simulink model "BatteryController_empat_PV_WindTurbine_fix1"  (R2015a)
settings: Solver=FixedStepDiscrete  StartTime=0.0  StopTime=10.0  FixedStep=5e-6  RelTol=1e-3
values from neighbouring files (symbols this model uses):
  n = 1500    [ini.m]
  Rs = 2.6e-3    (= 0.0026)    [ini.m]
undefined symbols (not defined in the file or in its folder): Eg0, Ion, Isc, K, ki, Lithium, Ns, q, Rsh, Tn, Voc
libraries: powerlib x56, electricdrivelib x5, re_lib x1
settings Model: Creator=Jodi  LastModifiedBy=David

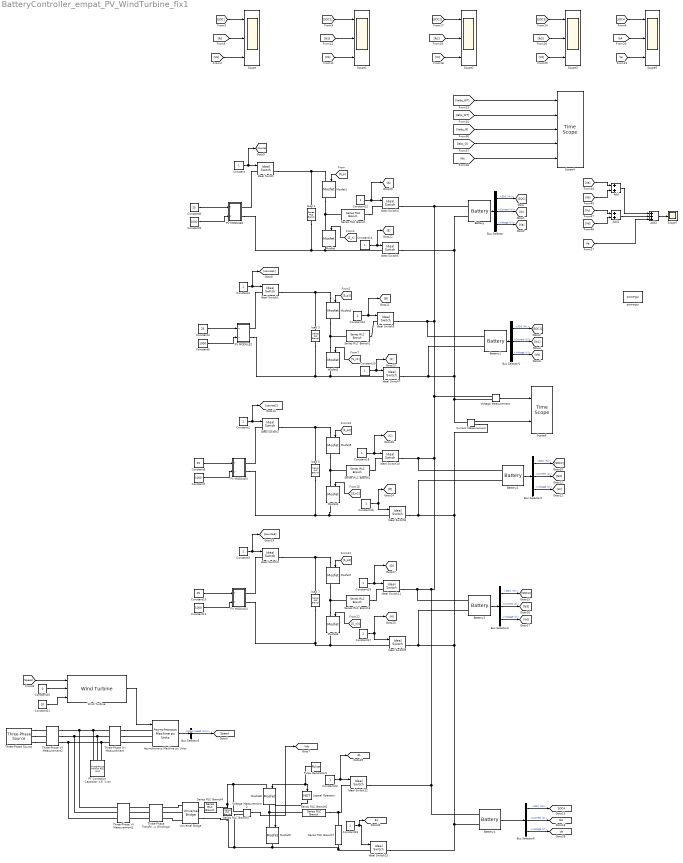
== system BatteryController_empat_PV_WindTurbine_fix1 ==
  Add : Sum
  Add1 : Sum
  Add2 : Sum  Inputs=+++
  Asynchronous Machine pu Units : powerlib/Machines/Asynchronous Machine pu Units  RotorType=Squirrel-cage  PresetModel=No  MechanicalLoad=Torque Tm  ShowDetailedParameters=on  ReferenceFrame=Rotor  Units=pu  MeasurementBus=off  NominalParameters=[400 220 50]  Stator=[0.01965 0.0397]  Rotor=[0.01909 0.0397]  Cage1=[0.01909 0.0397]  Cage2=[0.01909 0.0397]  Lm=1.354  Mechanical=[0.09526 0.05479 2]  PolePairs=2  InitialConditions="[ 1,0   0,0,0   0,0,0 ]"  SimulateSaturation=off  Saturation="[0.212,0.4201,0.8125,1.0979,1.4799,2.2457,3.2586,4.5763,6.4763 ;   0.5,0.7,0.9,1,1.1,1.2 ,1.3,1.4,1.5]"  LoadFlowParameters=0  TsPowergui=0  TsBlock=-1  IterativeModel=Trapezoidal non iterative  Pmec=0
  Battery{,1..3} (4 alike) : electricdrivelib/Extra Sources/Battery  BatType=Lithium-Ion  ShowDetailedParameters=off  NomV=12  NomQ=50  SOC=45  PresetModel=on  MaxQ=50  FullV=13.9678  Dis_rate=21.7391  R=0.0024  Normal_OP=45.2174  expZone="[12.9646      2.45652]"  current=[6.5 13 32.5]  Units=Time  Batt_Tr=1
  Battery4 : electricdrivelib/Extra Sources/Battery  BatType=Lithium-Ion  ShowDetailedParameters=off  NomV=12  NomQ=12  SOC=45  PresetModel=on  MaxQ=12  FullV=13.9678  Dis_rate=5.2174  R=0.01  Normal_OP=10.8522  expZone="[12.9646     0.589565]"  current=[6.5 13 32.5]  Units=Time  Batt_Tr=30
  Bus Selector{,1..3,6} (5 alike) : BusSelector  OutputSignals=SOC (%),Current (A),Voltage (V)
  Bus Selector5 : BusSelector  OutputSignals=Mechanical.Rotor speed (wm)
  Constant{,1..3,12..19,22..23} (14 alike) : Constant
  Constant{4,6,8,10} (4 alike) : Constant  Value=25
  Constant{5,7,9,11} (4 alike) : Constant  Value=1000
  Constant20 : Constant  Value=0
  Constant21 : Constant  Value=10
  Current Measurement : powerlib/Measurements/Current Measurement  PhasorSimulation=off  OutputType=Complex  PSBequivalent=0
  Ideal Switch{,1..13} (14 alike) : powerlib/Power Electronics/Ideal Switch  Ron=0.001  Lon=0  IC=0  Rs=1e5  Cs=inf  Measurements=on
  Logical Operator : Logic  Operator=NOT  AllPortsSameDT=off  OutDataTypeStr=boolean
  Mosfet{,1..7} (8 alike) : powerlib/Power Electronics/Mosfet  Ron=0.1  Lon=0  Rd=0.01  Vfd=0  IC=0  Rs=1e5  Cs=inf  Measurements=on
  Mosfet8 : powerlib/Power Electronics/Mosfet  Ron=0.1  Lon=0  Rd=0.01  Vfd=0  IC=0  Rs=1e5  Cs=inf  Measurements=off
  Mosfet9 : powerlib/Power Electronics/Mosfet  Ron=0.1  Lon=0  Rd=0.01  Vfd=0  IC=0  Rs=1e5  Cs=inf  Measurements=off
  PF Correction Capacitor 1.5  kvar : powerlib/Elements/Three-Phase Parallel RLC Load  LConnTagsString=A|B|C  Configuration=Delta  NominalVoltage=480  NominalFrequency=50  ActivePower=0  InductivePower=0  CapacitivePower=1.5e3  Measurements=None  LoadType=constant Z
  PV MODULE1 : Subsystem
  PV MODULE2 : Subsystem
  PV MODULE3 : Subsystem
  PV MODULE4 : Subsystem
  Pulse Generator3 : DiscretePulseGenerator  PulseType=Time based  Period=10  PulseWidth=5
  Scope{,1..3,5} (5 alike) : Scope  NumInputPorts=3
      Scope settings: TimeRange=10  YMin=42.75~-7.04708e-05~12.2718  YMax=47.25~-7.04704e-05~13.5636  SampleInput=on
      Scope1 settings: TimeRange=10  YMin=42.75~-0.00025~12.2718  YMax=47.25~0~13.5636  SampleInput=on
      Scope2 settings: TimeRange=10  YMin=42.75~0~24.5437  YMax=47.25~4e-05~27.1273  SaveName=ScopeData2  SampleInput=on
      Scope3 settings: TimeRange=10  YMin=42.75~0~24.5437  YMax=47.25~4e-05~27.1273  SaveName=ScopeData3  SampleInput=on
      Scope5 settings: TimeRange=10  YMin=0~-1~0  YMax=100~1~50  SaveName=ScopeData5  SampleInput=on
  Scope4 : TimeScope  NumInputPorts=5
  Scope6 : TimeScope  NumInputPorts=2
  Scope7 : Scope
      settings: YMin=0  YMax=70  SaveName=ScopeData7
  Series RLC Branch{,1..3} (4 alike) : powerlib/Elements/Series RLC Branch  LConnTagsString=__new0  RConnTagsString=__new0  BranchType=RL  Resistance=0.05  Inductance=5.76e-4  SetiL0=off  InitialCurrent=0  Capacitance=1e-6  Setx0=off  InitialVoltage=0  Measurements=None
  Series RLC Branch4 : powerlib/Elements/Series RLC Branch  LConnTagsString=__new0  RConnTagsString=__new0  BranchType=L  Resistance=100  Inductance=1e-3  SetiL0=off  InitialCurrent=0  Capacitance=1e-6  Setx0=off  InitialVoltage=0  Measurements=None
  Series RLC Branch5 : powerlib/Elements/Series RLC Branch  LConnTagsString=__new0  RConnTagsString=__new0  BranchType=C  Resistance=100  Inductance=1e-3  SetiL0=off  InitialCurrent=0  Capacitance=1e-3  Setx0=off  InitialVoltage=0  Measurements=None
  Series RLC Branch6 : powerlib/Elements/Series RLC Branch  LConnTagsString=__new0  RConnTagsString=__new0  BranchType=RL  Resistance=100  Inductance=1e-3  SetiL0=off  InitialCurrent=0  Capacitance=1e-6  Setx0=off  InitialVoltage=0  Measurements=None
  Series RLC Branch7 : powerlib/Elements/Series RLC Branch  LConnTagsString=__new0  RConnTagsString=__new0  BranchType=RC  Resistance=100  Inductance=1e-3  SetiL0=off  InitialCurrent=0  Capacitance=1e-6  Setx0=off  InitialVoltage=0  Measurements=None
  Three-Phase Transformer (Two Windings) : powerlib/Elements/Three-Phase Transformer (Two Windings)  Winding1Connection=Yg  Winding2Connection=Yg  CoreType=Three single-phase transformers  SetSaturation=off  Hysteresis=off  DataFile='hysteresis'  SetInitialFlux=off  Measurements=None  UNITS=pu  NominalPower=[ 250e6 , 50 ]  Winding1=[ 735e3 , 0.002 , 0.08 ]  Winding2=[ 315e3 , 0.002 , 0.08 ]  Rm=100  Lm=500  L0=0.5  Saturation=[ 0,0 ; 0.0024,1.2 ; 1.0,1.52 ]  InitialFluxes=[ 0.8 , -0.8 , 0.7 ]  MoreParameters=off  BreakLoop=off  DataType=off  TransfoNumber=1
  Three-Phase V-I Measurement : powerlib/Measurements/Three-Phase V-I Measurement  VoltageMeasurement=phase-to-ground  SetLabelV=on  LabelV=Vabc_WT  Vpu=off  VpuLL=off  CurrentMeasurement=yes  SetLabelI=on  LabelI=Iabc_WT  Ipu=off  Pbase=100e6  Vbase=500e3  OutputType=Complex  PhasorSimulation=off  PSBequivalent=0
  Three-Phase V-I Measurement1 : powerlib/Measurements/Three-Phase V-I Measurement  VoltageMeasurement=phase-to-phase  SetLabelV=on  LabelV=Vabc_G  Vpu=off  VpuLL=off  CurrentMeasurement=yes  SetLabelI=on  LabelI=Iabc_G  Ipu=off  Pbase=100e6  Vbase=500e3  OutputType=Complex  PhasorSimulation=off  PSBequivalent=0
  Three-Phase V-I Measurement2 : powerlib/Measurements/Three-Phase V-I Measurement  VoltageMeasurement=phase-to-ground  SetLabelV=on  LabelV=Vabc_SC  Vpu=off  VpuLL=off  CurrentMeasurement=yes  SetLabelI=on  LabelI=Iabc_SC  Ipu=off  Pbase=100e6  Vbase=500e3  OutputType=Complex  PhasorSimulation=off  PSBequivalent=0
  Three-Phase Source : powerlib/Electrical Sources/Three-Phase Source  Voltage=220  PhaseAngle=4  Frequency=50  InternalConnection=Yg  SpecifyImpedance=on  Resistance=0.8929  Inductance=16.58e-3  ShortCircuitLevel=100e6  BaseVoltage=25e3  XRratio=7  BusType=swing  Pref=0  Qref=0  Qmin=-inf  Qmax=inf
  Universal Bridge : powerlib/Power Electronics/Universal Bridge  Arms=3  SnubberResistance=100  SnubberCapacitance=inf  Device=Diodes  Ron=1e-3  Lon=0  ForwardVoltages="[  0  0  ]"  ForwardVoltage=0  GTOparameters=[ 10e-6 , 20e-6 ]  IGBTparameters=[ 1e-6 , 2e-6 ]  Measurements=None  Measurements_2=None  converterType=Rectifier
  Voltage Measurement : powerlib/Measurements/Voltage Measurement  PhasorSimulation=off  OutputType=Complex  PSBequivalent=0
  Voltage Measurement2 : powerlib/Measurements/Voltage Measurement  PhasorSimulation=off  OutputType=Complex  PSBequivalent=0
  Wind Turbine : re_lib/Wind Generation/Wind Turbine  Pnom=400  Pelec_base=400/0.9  wind_base=12  P_wind_base=0.73  speed_nom=1.2  pitch_angle=0  c1_c6="[0.51763          116          0.4            5           21     0.006795]"  cp_nom=0.48  lambda_nom=8.1
  load {1,3,5,7} (4 alike) : powerlib/Elements/Series RLC Branch  LConnTagsString=__new0  RConnTagsString=__new0  BranchType=RC  Resistance=0.001  Inductance=5.76e-4  SetiL0=off  InitialCurrent=0  Capacitance=1000e-6  Setx0=off  InitialVoltage=0  Measurements=None
  powergui : powerlib/powergui  Priority=1  SimulationMode=Discrete  SolverType=Tustin/Backward Euler (TBE)  SampleTime=5e-06  frequency=60  SPID=off  DisableSnubberDevices=off  DisableRonSwitches=off  DisableVfSwitches=off  SwTol=0  DisplayEquations=off  Interpol=off  methode=off  Ts=100  FunctionMessages=off  echomessages=off  HookPort=off  EnableUseOfTLC=off  x0status=blocks  frequencyindice=0  Pbase=100e6  ErrMax=1e-4  Iterations=50  UnitsV=kV  UnitsW=MW  buscounter=0  RestoreLinks=warning  ResistiveCurrentMeasurement=off  Frange=[0:2:500]  Ylog=off  Xlog=on  ShowGrid=off  save=off  variable=ZData  structure=0  ZoomFFT=off  StartTime=0.0  cycles=1  DisplayStyle=1  fundamental=60  FreqAxis=off  MaxFrequency=1000  frequencyindicesteady=1  RmsSteady=1  display=off
  tag scope: A1=global, E1=global, Ib4=global, SOC4=global, Speed=global, Vdc=global, Ve=global
  wires:
  Constant/1 -> [source], Ideal Switch/1
  Battery/1 -> Bus Selector/1
  Bus Selector/1 -> [SOC]  "<SOC (%)>"
  Bus Selector/2 -> [Ib]  "<Current (A)>"
  Bus Selector/3 -> [Va]  "<Voltage (V)>"
  [S_p] -> Mosfet1/1
  [S_n] -> Mosfet/1
  [SOC] -> Scope/1
  [Va] -> Scope/3
  Constant1/1 -> [source1], Ideal Switch1/1
  Battery1/1 -> Bus Selector1/1
  Bus Selector1/1 -> [SOC1]  "<SOC (%)>"
  Bus Selector1/2 -> [Ib1]  "<Current (A)>"
  Bus Selector1/3 -> [Vb]  "<Voltage (V)>"
  [S_p1] -> Mosfet3/1
  [S_n1] -> Mosfet2/1
  [SOC1] -> Scope1/1
  [Vb] -> Scope1/3
  Constant2/1 -> [source2], Ideal Switch2/1
  Battery2/1 -> Bus Selector2/1
  Bus Selector2/1 -> [SOC2]  "<SOC (%)>"
  Bus Selector2/2 -> [Ib2]  "<Current (A)>"
  Bus Selector2/3 -> [Vc]  "<Voltage (V)>"
  [S_p2] -> Mosfet5/1
  [S_n2] -> Mosfet4/1
  [SOC2] -> Scope2/1
  [Vc] -> Scope2/3
  Constant3/1 -> [source3], Ideal Switch3/1
  Battery3/1 -> Bus Selector3/1
  Bus Selector3/1 -> [SOC3]  "<SOC (%)>"
  Bus Selector3/2 -> [Ib3]  "<Current (A)>"
  Bus Selector3/3 -> [Vd]  "<Voltage (V)>"
  [S_p3] -> Mosfet7/1
  [S_n3] -> Mosfet6/1
  [SOC3] -> Scope3/1
  [Vd] -> Scope3/3
  Constant8/1 -> PV MODULE1/1(T)
  Constant9/1 -> PV MODULE1/2(Ir)
  Constant4/1 -> PV MODULE2/1(T)
  Constant5/1 -> PV MODULE2/2(Ir)
  Constant6/1 -> PV MODULE3/1(T)
  Constant7/1 -> PV MODULE3/2(Ir)
  Constant10/1 -> PV MODULE4/1(T)
  Constant11/1 -> PV MODULE4/2(Ir)
  Constant12/1 -> [A], Ideal Switch4/1
  Constant13/1 -> [B], Ideal Switch5/1
  Constant14/1 -> [E], Ideal Switch6/1
  Constant15/1 -> Ideal Switch7/1, [F]
  Constant16/1 -> [G], Ideal Switch8/1
  Constant17/1 -> [H], Ideal Switch9/1
  Constant18/1 -> [C], Ideal Switch10/1
  Constant19/1 -> [D], Ideal Switch11/1
  Wind Turbine/1 -> Asynchronous Machine pu Units/1
  Asynchronous Machine pu Units/1 -> Bus Selector5/1
  Bus Selector5/1 -> [Speed]  "<Rotor speed (wm)>"
  [Speed] -> Wind Turbine/1
  Constant20/1 -> Wind Turbine/2
  Constant21/1 -> Wind Turbine/3
  Battery4/1 -> Bus Selector6/1
  Pulse Generator3/1 -> Logical Operator/1, Mosfet8/1
  Logical Operator/1 -> Mosfet9/1
  Voltage Measurement2/1 -> [Vdc]
  Bus Selector6/1 -> [SOC4]  "<SOC (%)>"
  Bus Selector6/2 -> [Ib4]  "<Current (A)>"
  Bus Selector6/3 -> [Ve]  "<Voltage (V)>"
  [Vabc_WT] -> Scope4/1
  [Iabc_G] -> Scope4/4
  [Vabc_G] -> Scope4/3
  [Iabc_WT] -> Scope4/2
  [Vdc] -> Scope4/5
  Constant22/1 -> [A1], Ideal Switch12/1
  Constant23/1 -> [E1], Ideal Switch13/1
  [Ib] -> Scope/2
  [Ib1] -> Scope1/2
  [Ib2] -> Scope2/2
  [Ib3] -> Scope3/2
  [SOC4] -> Scope5/1
  [Ve] -> Scope5/3
  [Ib4] -> Scope5/2
  [Va] -> Add/1
  [Vb] -> Add/2
  [Vc] -> Add1/1
  [Vd] -> Add1/2
  Add/1 -> Add2/1
  Add1/1 -> Add2/2
  Add2/1 -> Scope7/1
  [Ve] -> Add2/3
  Current Measurement/1 -> Scope6/2
  Voltage Measurement/1 -> Scope6/1
  connections:
  Mosfet1/RConn1 -- Series RLC Branch/LConn1 -- Mosfet/LConn1
  PV MODULE1/RConn2 -- load 1/RConn1 -- Ideal Switch6/LConn1 -- Mosfet/RConn1
  load 1/LConn1 -- Ideal Switch/RConn1 -- Mosfet1/LConn1
  Ideal Switch/LConn1 -- PV MODULE1/RConn1
  Mosfet2/LConn1 -- Mosfet3/RConn1 -- Series RLC Branch1/LConn1
  load 3/RConn1 -- PV MODULE2/RConn2 -- Mosfet2/RConn1 -- Ideal Switch7/LConn1
  Mosfet3/LConn1 -- Ideal Switch1/RConn1 -- load 3/LConn1
  Ideal Switch1/LConn1 -- PV MODULE2/RConn1
  Mosfet4/LConn1 -- Mosfet5/RConn1 -- Series RLC Branch2/LConn1
  load 5/RConn1 -- PV MODULE3/RConn2 -- Mosfet4/RConn1 -- Ideal Switch8/LConn1
  Mosfet5/LConn1 -- Ideal Switch2/RConn1 -- load 5/LConn1
  Ideal Switch2/LConn1 -- PV MODULE3/RConn1
  Mosfet6/LConn1 -- Mosfet7/RConn1 -- Series RLC Branch3/LConn1
  load 7/RConn1 -- PV MODULE4/RConn2 -- Ideal Switch9/LConn1 -- Mosfet6/RConn1
  Mosfet7/LConn1 -- Ideal Switch3/RConn1 -- load 7/LConn1
  Ideal Switch3/LConn1 -- PV MODULE4/RConn1
  Series RLC Branch/RConn1 -- Ideal Switch4/LConn1
  Ideal Switch5/LConn1 -- Series RLC Branch1/RConn1
  Series RLC Branch2/RConn1 -- Ideal Switch10/LConn1
  Series RLC Branch3/RConn1 -- Ideal Switch11/LConn1
  PF Correction Capacitor 1.5  kvar/LConn1 -- Three-Phase V-I Measurement/RConn1 -- Three-Phase V-I Measurement1/LConn1 -- Three-Phase V-I Measurement2/RConn1
  PF Correction Capacitor 1.5  kvar/LConn2 -- Three-Phase V-I Measurement/RConn2 -- Three-Phase V-I Measurement1/LConn2 -- Three-Phase V-I Measurement2/RConn2
  PF Correction Capacitor 1.5  kvar/LConn3 -- Three-Phase V-I Measurement/RConn3 -- Three-Phase V-I Measurement1/LConn3 -- Three-Phase V-I Measurement2/RConn3
  Series RLC Branch5/LConn1 -- Voltage Measurement2/LConn1 -- Mosfet8/LConn1 -- Series RLC Branch4/RConn1
  Series RLC Branch6/LConn1 -- Mosfet8/RConn1 -- Mosfet9/LConn1
  Series RLC Branch5/RConn1 -- Ideal Switch13/LConn1 -- Series RLC Branch7/RConn1 -- Mosfet9/RConn1 -- Voltage Measurement2/LConn2 -- Universal Bridge/RConn2
  Three-Phase V-I Measurement/LConn1 -- Asynchronous Machine pu Units/LConn1
  Three-Phase V-I Measurement/LConn3 -- Asynchronous Machine pu Units/LConn3
  Three-Phase V-I Measurement/LConn2 -- Asynchronous Machine pu Units/LConn2
  Universal Bridge/LConn3 -- Three-Phase Transformer (Two Windings)/RConn3
  Three-Phase Transformer (Two Windings)/LConn2 -- Three-Phase V-I Measurement1/RConn2
  Universal Bridge/LConn1 -- Three-Phase Transformer (Two Windings)/RConn1
  Three-Phase Transformer (Two Windings)/LConn1 -- Three-Phase V-I Measurement1/RConn1
  Universal Bridge/LConn2 -- Three-Phase Transformer (Two Windings)/RConn2
  Series RLC Branch4/LConn1 -- Universal Bridge/RConn1
  Three-Phase Transformer (Two Windings)/LConn3 -- Three-Phase V-I Measurement1/RConn3
  Series RLC Branch6/RConn1 -- Series RLC Branch7/LConn1 -- Ideal Switch12/LConn1
  Three-Phase Source/RConn1 -- Three-Phase V-I Measurement2/LConn1
  Three-Phase Source/RConn2 -- Three-Phase V-I Measurement2/LConn2
  Three-Phase Source/RConn3 -- Three-Phase V-I Measurement2/LConn3
  Battery4/LConn1 -- Ideal Switch12/RConn1 -- Battery3/LConn1 -- Ideal Switch11/RConn1 -- Battery2/LConn1 -- Ideal Switch10/RConn1 -- Ideal Switch5/RConn1 -- Battery1/LConn1 -- Ideal Switch4/RConn1 -- Battery/LConn1 -- Voltage Measurement/LConn1
  Battery/LConn2 -- Ideal Switch6/RConn1 -- Ideal Switch7/RConn1 -- Battery1/LConn2 -- Current Measurement/LConn1 -- Voltage Measurement/LConn2
  Ideal Switch13/RConn1 -- Battery3/LConn2 -- Ideal Switch9/RConn1 -- Battery2/LConn2 -- Ideal Switch8/RConn1 -- Current Measurement/RConn1 -- Battery4/LConn2

== system BatteryController_empat_PV_WindTurbine_fix1/PV MODULE1 ==
  T : Inport
  Ir : Inport  Port=2
  Controlled Current Source : powerlib/Electrical Sources/Controlled Current Source  Initialize=on  Source_Type=AC  Amplitude=0  Phase=0  Frequency=0  Measurements=None
  PV Module : Subsystem  InitFcn=|
      | ki=.0032,
      | q=1.6e-19,
      | K=1.38e-23,
      | n=1.3,
      | Eg0=1.1,
      | Rs=.221,
      | Rsh=415.405,
      | Tn=298,
      | 
      | Voc=32.9,
      | Isc=8.21,
      | Ns=54,
  Voltage Measurement : powerlib/Measurements/Voltage Measurement  PhasorSimulation=off  OutputType=Complex  PSBequivalent=0
  + : PMIOPort  Port=1  Side=Right
  - : PMIOPort  Port=2  Side=Right
  wires:
  Voltage Measurement/1 -> PV Module/3(V_Array)
  PV Module/1(I) -> Controlled Current Source/1
  Ir/1 -> PV Module/2(G)
  T/1 -> PV Module/1(T)
  connections:
  Controlled Current Source/RConn1 -- +/RConn1 -- Voltage Measurement/LConn1
  Controlled Current Source/LConn1 -- -/RConn1 -- Voltage Measurement/LConn2

== system BatteryController_empat_PV_WindTurbine_fix1/PV MODULE2 ==
  T : Inport
  Ir : Inport  Port=2
  Controlled Current Source : powerlib/Electrical Sources/Controlled Current Source  Initialize=on  Source_Type=AC  Amplitude=0  Phase=0  Frequency=0  Measurements=None
  PV Module : Subsystem  InitFcn=|
      | ki=.0032,
      | q=1.6e-19,
      | K=1.38e-23,
      | n=1.3,
      | Eg0=1.1,
      | Rs=.221,
      | Rsh=415.405,
      | Tn=298,
      | 
      | Voc=32.9,
      | Isc=8.21,
      | Ns=54,
  Voltage Measurement : powerlib/Measurements/Voltage Measurement  PhasorSimulation=off  OutputType=Complex  PSBequivalent=0
  + : PMIOPort  Port=1  Side=Right
  - : PMIOPort  Port=2  Side=Right
  wires:
  Voltage Measurement/1 -> PV Module/3(V_Array)
  PV Module/1(I) -> Controlled Current Source/1
  Ir/1 -> PV Module/2(G)
  T/1 -> PV Module/1(T)
  connections:
  Controlled Current Source/RConn1 -- +/RConn1 -- Voltage Measurement/LConn1
  Controlled Current Source/LConn1 -- -/RConn1 -- Voltage Measurement/LConn2

== system BatteryController_empat_PV_WindTurbine_fix1/PV MODULE3 ==
  T : Inport
  Ir : Inport  Port=2
  Controlled Current Source : powerlib/Electrical Sources/Controlled Current Source  Initialize=on  Source_Type=AC  Amplitude=0  Phase=0  Frequency=0  Measurements=None
  PV Module : Subsystem  InitFcn=|
      | ki=.0032,
      | q=1.6e-19,
      | K=1.38e-23,
      | n=1.3,
      | Eg0=1.1,
      | Rs=.221,
      | Rsh=415.405,
      | Tn=298,
      | 
      | Voc=32.9,
      | Isc=8.21,
      | Ns=54,
  Voltage Measurement : powerlib/Measurements/Voltage Measurement  PhasorSimulation=off  OutputType=Complex  PSBequivalent=0
  + : PMIOPort  Port=1  Side=Right
  - : PMIOPort  Port=2  Side=Right
  wires:
  Voltage Measurement/1 -> PV Module/3(V_Array)
  PV Module/1(I) -> Controlled Current Source/1
  Ir/1 -> PV Module/2(G)
  T/1 -> PV Module/1(T)
  connections:
  Controlled Current Source/RConn1 -- +/RConn1 -- Voltage Measurement/LConn1
  Controlled Current Source/LConn1 -- -/RConn1 -- Voltage Measurement/LConn2

== system BatteryController_empat_PV_WindTurbine_fix1/PV MODULE4 ==
  T : Inport
  Ir : Inport  Port=2
  Controlled Current Source : powerlib/Electrical Sources/Controlled Current Source  Initialize=on  Source_Type=AC  Amplitude=0  Phase=0  Frequency=0  Measurements=None
  PV Module : Subsystem  InitFcn=|
      | ki=.0032,
      | q=1.6e-19,
      | K=1.38e-23,
      | n=1.3,
      | Eg0=1.1,
      | Rs=.221,
      | Rsh=415.405,
      | Tn=298,
      | 
      | Voc=32.9,
      | Isc=8.21,
      | Ns=54,
  Voltage Measurement : powerlib/Measurements/Voltage Measurement  PhasorSimulation=off  OutputType=Complex  PSBequivalent=0
  + : PMIOPort  Port=1  Side=Right
  - : PMIOPort  Port=2  Side=Right
  wires:
  Voltage Measurement/1 -> PV Module/3(V_Array)
  PV Module/1(I) -> Controlled Current Source/1
  Ir/1 -> PV Module/2(G)
  T/1 -> PV Module/1(T)
  connections:
  Controlled Current Source/RConn1 -- +/RConn1 -- Voltage Measurement/LConn1
  Controlled Current Source/LConn1 -- -/RConn1 -- Voltage Measurement/LConn2

== system BatteryController_empat_PV_WindTurbine_fix1/PV MODULE1/PV Module ==
  T : Inport
  G : Inport  Port=2
  V_Array : Inport  Port=3
  Add1 : Sum
  Constant1 : Constant  Value=273
  Photo Current : Subsystem
  Pv Current : Subsystem
  Reverse Saturation Current : Subsystem
  Saturation Current : Subsystem
  Shunt Current : Subsystem
  I : Outport
  wires:
  Pv Current/1(I) -> I/1, Shunt Current/2(I)
  Photo Current/1(Iph) -> Pv Current/4(Iph)
  Saturation Current/1(IO) -> Pv Current/3(IO)
  V_Array/1 -> Shunt Current/1(V), Pv Current/1(V)
  T/1 -> Add1/1
  G/1 -> Photo Current/2(G)
  Reverse Saturation Current/1(Irs) -> Saturation Current/2(Irs)
  Shunt Current/1(Ish) -> Pv Current/5(Ish)
  Constant1/1 -> Add1/2
  Add1/1 -> Saturation Current/1(T), Photo Current/1(T), Reverse Saturation Current/1(T), Pv Current/2(T)

== system BatteryController_empat_PV_WindTurbine_fix1/PV MODULE2/PV Module ==
  T : Inport
  G : Inport  Port=2
  V_Array : Inport  Port=3
  Add1 : Sum
  Constant1 : Constant  Value=273
  Photo Current : Subsystem
  Pv Current : Subsystem
  Reverse Saturation Current : Subsystem
  Saturation Current : Subsystem
  Shunt Current : Subsystem
  I : Outport
  wires:
  Pv Current/1(I) -> I/1, Shunt Current/2(I)
  Photo Current/1(Iph) -> Pv Current/4(Iph)
  Saturation Current/1(IO) -> Pv Current/3(IO)
  V_Array/1 -> Shunt Current/1(V), Pv Current/1(V)
  T/1 -> Add1/1
  G/1 -> Photo Current/2(G)
  Reverse Saturation Current/1(Irs) -> Saturation Current/2(Irs)
  Shunt Current/1(Ish) -> Pv Current/5(Ish)
  Constant1/1 -> Add1/2
  Add1/1 -> Saturation Current/1(T), Photo Current/1(T), Reverse Saturation Current/1(T), Pv Current/2(T)

== system BatteryController_empat_PV_WindTurbine_fix1/PV MODULE3/PV Module ==
  T : Inport
  G : Inport  Port=2
  V_Array : Inport  Port=3
  Add1 : Sum
  Constant1 : Constant  Value=273
  Photo Current : Subsystem
  Pv Current : Subsystem
  Reverse Saturation Current : Subsystem
  Saturation Current : Subsystem
  Shunt Current : Subsystem
  I : Outport
  wires:
  Pv Current/1(I) -> I/1, Shunt Current/2(I)
  Photo Current/1(Iph) -> Pv Current/4(Iph)
  Saturation Current/1(IO) -> Pv Current/3(IO)
  V_Array/1 -> Shunt Current/1(V), Pv Current/1(V)
  T/1 -> Add1/1
  G/1 -> Photo Current/2(G)
  Reverse Saturation Current/1(Irs) -> Saturation Current/2(Irs)
  Shunt Current/1(Ish) -> Pv Current/5(Ish)
  Constant1/1 -> Add1/2
  Add1/1 -> Saturation Current/1(T), Photo Current/1(T), Reverse Saturation Current/1(T), Pv Current/2(T)

== system BatteryController_empat_PV_WindTurbine_fix1/PV MODULE4/PV Module ==
  T : Inport
  G : Inport  Port=2
  V_Array : Inport  Port=3
  Add1 : Sum
  Constant1 : Constant  Value=273
  Photo Current : Subsystem
  Pv Current : Subsystem
  Reverse Saturation Current : Subsystem
  Saturation Current : Subsystem
  Shunt Current : Subsystem
  I : Outport
  wires:
  Pv Current/1(I) -> I/1, Shunt Current/2(I)
  Photo Current/1(Iph) -> Pv Current/4(Iph)
  Saturation Current/1(IO) -> Pv Current/3(IO)
  V_Array/1 -> Shunt Current/1(V), Pv Current/1(V)
  T/1 -> Add1/1
  G/1 -> Photo Current/2(G)
  Reverse Saturation Current/1(Irs) -> Saturation Current/2(Irs)
  Shunt Current/1(Ish) -> Pv Current/5(Ish)
  Constant1/1 -> Add1/2
  Add1/1 -> Saturation Current/1(T), Photo Current/1(T), Reverse Saturation Current/1(T), Pv Current/2(T)

== system BatteryController_empat_PV_WindTurbine_fix1/PV MODULE1/PV Module/Photo Current ==
  note: Iph=[Isc + {ki*(T-298)}]*G/1000
  T : Inport
  G : Inport  Port=2
  Add1 : Sum  Inputs=+-
  Add2 : Sum  Inputs=+-
  Constant1 : Constant  Value=298
  Constant2 : Constant  Value=ki
  Constant3 : Constant  Value=Isc
  Constant4 : Constant  Value=1000
  Product1 : Product
  Product2 : Product
  Product3 : Product  Inputs=*/
  Iph : Outport
  wires:
  Add2/1 -> Product2/2
  Product3/1 -> Iph/1
  Constant4/1 -> Product3/2
  Constant1/1 -> Add1/2
  Product2/1 -> Product3/1
  G/1 -> Product2/1
  Constant2/1 -> Product1/2
  Product1/1 -> Add2/2
  Add1/1 -> Product1/1
  T/1 -> Add1/1
  Constant3/1 -> Add2/1

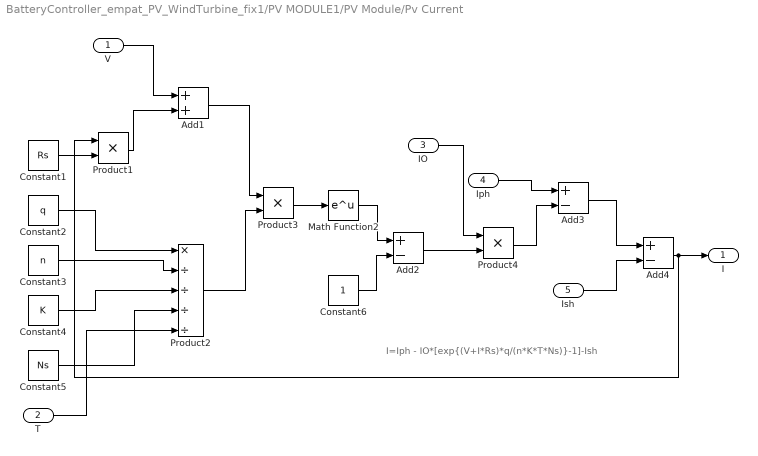
== system BatteryController_empat_PV_WindTurbine_fix1/PV MODULE1/PV Module/Pv Current ==
  note: I=Iph - IO*[exp{(V+I*Rs)*q/(n*K*T*Ns)}-1]-Ish
  V : Inport
  T : Inport  Port=2
  IO : Inport  Port=3
  Iph : Inport  Port=4
  Ish : Inport  Port=5
  Add1 : Sum
  Add2 : Sum  Inputs=+-
  Add3 : Sum  Inputs=+-
  Add4 : Sum  Inputs=+-
  Constant1 : Constant  Value=Rs
  Constant2 : Constant  Value=q
  Constant3 : Constant  Value=n
  Constant4 : Constant  Value=K
  Constant5 : Constant  Value=Ns
  Constant6 : Constant
  Math Function2 : Math  SaturateOnIntegerOverflow=on
  Product1 : Product
  Product2 : Product  Inputs=*////
  Product3 : Product
  Product4 : Product
  I : Outport
  wires:
  Constant3/1 -> Product2/2
  Constant4/1 -> Product2/3
  Add2/1 -> Product4/2
  Add3/1 -> Add4/1
  Constant5/1 -> Product2/4
  Iph/1 -> Add3/1
  Product1/1 -> Add1/2
  Product2/1 -> Product3/2
  T/1 -> Product2/5
  Product3/1 -> Math Function2/1
  Math Function2/1 -> Add2/1
  Add1/1 -> Product3/1
  Constant2/1 -> Product2/1
  V/1 -> Add1/1
  IO/1 -> Product4/1
  Constant6/1 -> Add2/2
  Ish/1 -> Add4/2
  Add4/1 -> I/1, Product1/1
  Product4/1 -> Add3/2
  Constant1/1 -> Product1/2

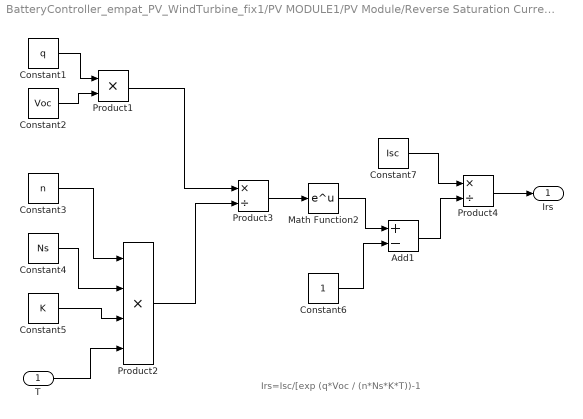
== system BatteryController_empat_PV_WindTurbine_fix1/PV MODULE1/PV Module/Reverse Saturation Current ==
  note: Irs=Isc/[exp (q*Voc / (n*Ns*K*T))-1
  T : Inport
  Add1 : Sum  Inputs=+-
  Constant1 : Constant  Value=q
  Constant2 : Constant  Value=Voc
  Constant3 : Constant  Value=n
  Constant4 : Constant  Value=Ns
  Constant5 : Constant  Value=K
  Constant6 : Constant
  Constant7 : Constant  Value=Isc
  Math Function2 : Math  SaturateOnIntegerOverflow=on
  Product1 : Product
  Product2 : Product  Inputs=4
  Product3 : Product  Inputs=*/
  Product4 : Product  Inputs=*/
  Irs : Outport
  wires:
  Product4/1 -> Irs/1
  Constant1/1 -> Product1/1
  Math Function2/1 -> Add1/1
  Constant6/1 -> Add1/2
  Constant3/1 -> Product2/1
  Add1/1 -> Product4/2
  Product2/1 -> Product3/2
  Constant7/1 -> Product4/1
  Product3/1 -> Math Function2/1
  Product1/1 -> Product3/1
  Constant2/1 -> Product1/2
  T/1 -> Product2/4
  Constant5/1 -> Product2/3
  Constant4/1 -> Product2/2

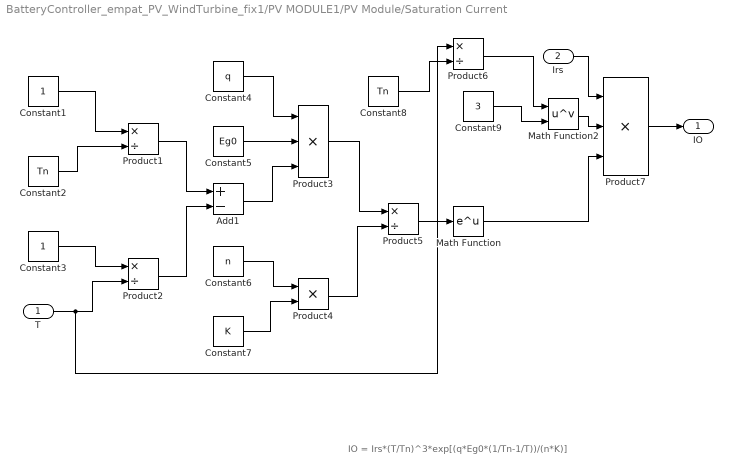
== system BatteryController_empat_PV_WindTurbine_fix1/PV MODULE1/PV Module/Saturation Current ==
  note: IO = Irs*(T/Tn)^3*exp[(q*Eg0*(1/Tn-1/T))/(n*K)]
  T : Inport
  Irs : Inport  Port=2
  Add1 : Sum  Inputs=+-
  Constant1 : Constant
  Constant2 : Constant  Value=Tn
  Constant3 : Constant
  Constant4 : Constant  Value=q
  Constant5 : Constant  Value=Eg0
  Constant6 : Constant  Value=n
  Constant7 : Constant  Value=K
  Constant8 : Constant  Value=Tn
  Constant9 : Constant  Value=3
  Math Function : Math  SaturateOnIntegerOverflow=on
  Math Function2 : Math  Operator=pow  SaturateOnIntegerOverflow=on
  Product{1..2,5..6} (4 alike) : Product  Inputs=*/
  Product3 : Product  Inputs=3
  Product4 : Product
  Product7 : Product  Inputs=3
  IO : Outport
  wires:
  Product7/1 -> IO/1
  Product4/1 -> Product5/2
  Product5/1 -> Math Function/1
  Math Function2/1 -> Product7/2
  Constant2/1 -> Product1/2
  Add1/1 -> Product3/3
  Constant5/1 -> Product3/2
  Constant7/1 -> Product4/2
  Constant4/1 -> Product3/1
  Constant8/1 -> Product6/2
  Product2/1 -> Add1/2
  T/1 -> Product6/1, Product2/2
  Constant1/1 -> Product1/1
  Math Function/1 -> Product7/3
  Product6/1 -> Math Function2/1
  Constant9/1 -> Math Function2/2
  Irs/1 -> Product7/1
  Constant3/1 -> Product2/1
  Product3/1 -> Product5/1
  Constant6/1 -> Product4/1
  Product1/1 -> Add1/1

== system BatteryController_empat_PV_WindTurbine_fix1/PV MODULE1/PV Module/Shunt Current ==
  note: Ish=(V+I*Rs)/Rsh
  V : Inport
  I : Inport  Port=2
  Add1 : Sum
  Constant1 : Constant  Value=Rs
  Constant2 : Constant  Value=Rsh
  Product1 : Product  Inputs=**
  Product2 : Product  Inputs=*/
  Ish : Outport
  wires:
  I/1 -> Product1/1
  Constant1/1 -> Product1/2
  Constant2/1 -> Product2/2
  Add1/1 -> Product2/1
  Product1/1 -> Add1/1
  Product2/1 -> Ish/1
  V/1 -> Add1/2

== system BatteryController_empat_PV_WindTurbine_fix1/PV MODULE2/PV Module/Photo Current ==
  note: Iph=[Isc + {ki*(T-298)}]*G/1000
  T : Inport
  G : Inport  Port=2
  Add1 : Sum  Inputs=+-
  Add2 : Sum  Inputs=+-
  Constant1 : Constant  Value=298
  Constant2 : Constant  Value=ki
  Constant3 : Constant  Value=Isc
  Constant4 : Constant  Value=1000
  Product1 : Product
  Product2 : Product
  Product3 : Product  Inputs=*/
  Iph : Outport
  wires:
  Add2/1 -> Product2/2
  Product3/1 -> Iph/1
  Constant4/1 -> Product3/2
  Constant1/1 -> Add1/2
  Product2/1 -> Product3/1
  G/1 -> Product2/1
  Constant2/1 -> Product1/2
  Product1/1 -> Add2/2
  Add1/1 -> Product1/1
  T/1 -> Add1/1
  Constant3/1 -> Add2/1

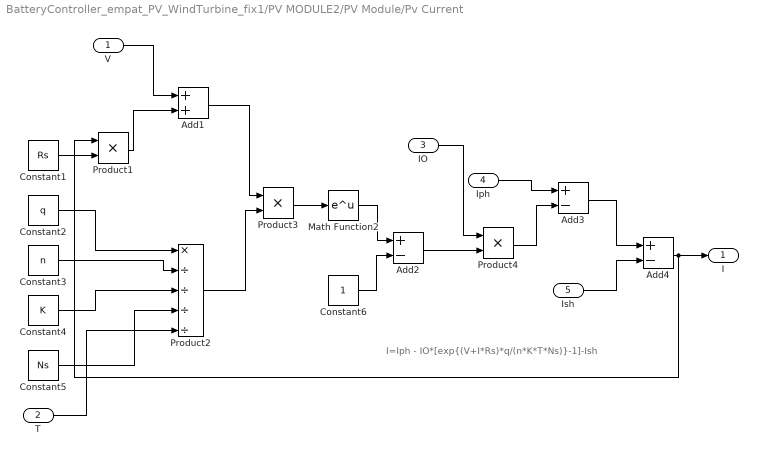
== system BatteryController_empat_PV_WindTurbine_fix1/PV MODULE2/PV Module/Pv Current ==
  note: I=Iph - IO*[exp{(V+I*Rs)*q/(n*K*T*Ns)}-1]-Ish
  V : Inport
  T : Inport  Port=2
  IO : Inport  Port=3
  Iph : Inport  Port=4
  Ish : Inport  Port=5
  Add1 : Sum
  Add2 : Sum  Inputs=+-
  Add3 : Sum  Inputs=+-
  Add4 : Sum  Inputs=+-
  Constant1 : Constant  Value=Rs
  Constant2 : Constant  Value=q
  Constant3 : Constant  Value=n
  Constant4 : Constant  Value=K
  Constant5 : Constant  Value=Ns
  Constant6 : Constant
  Math Function2 : Math  SaturateOnIntegerOverflow=on
  Product1 : Product
  Product2 : Product  Inputs=*////
  Product3 : Product
  Product4 : Product
  I : Outport
  wires:
  Constant3/1 -> Product2/2
  Constant4/1 -> Product2/3
  Add2/1 -> Product4/2
  Add3/1 -> Add4/1
  Constant5/1 -> Product2/4
  Iph/1 -> Add3/1
  Product1/1 -> Add1/2
  Product2/1 -> Product3/2
  T/1 -> Product2/5
  Product3/1 -> Math Function2/1
  Math Function2/1 -> Add2/1
  Add1/1 -> Product3/1
  Constant2/1 -> Product2/1
  V/1 -> Add1/1
  IO/1 -> Product4/1
  Constant6/1 -> Add2/2
  Ish/1 -> Add4/2
  Add4/1 -> I/1, Product1/1
  Product4/1 -> Add3/2
  Constant1/1 -> Product1/2

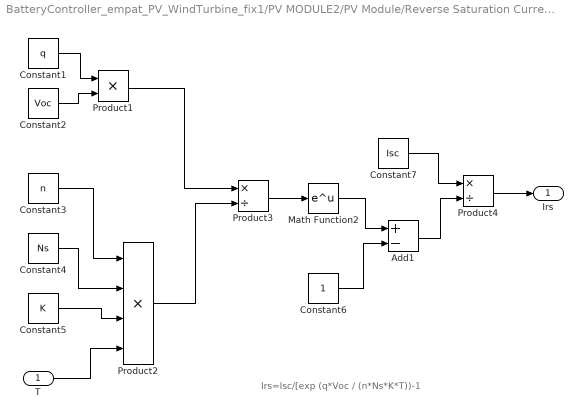
== system BatteryController_empat_PV_WindTurbine_fix1/PV MODULE2/PV Module/Reverse Saturation Current ==
  note: Irs=Isc/[exp (q*Voc / (n*Ns*K*T))-1
  T : Inport
  Add1 : Sum  Inputs=+-
  Constant1 : Constant  Value=q
  Constant2 : Constant  Value=Voc
  Constant3 : Constant  Value=n
  Constant4 : Constant  Value=Ns
  Constant5 : Constant  Value=K
  Constant6 : Constant
  Constant7 : Constant  Value=Isc
  Math Function2 : Math  SaturateOnIntegerOverflow=on
  Product1 : Product
  Product2 : Product  Inputs=4
  Product3 : Product  Inputs=*/
  Product4 : Product  Inputs=*/
  Irs : Outport
  wires:
  Product4/1 -> Irs/1
  Constant1/1 -> Product1/1
  Math Function2/1 -> Add1/1
  Constant6/1 -> Add1/2
  Constant3/1 -> Product2/1
  Add1/1 -> Product4/2
  Product2/1 -> Product3/2
  Constant7/1 -> Product4/1
  Product3/1 -> Math Function2/1
  Product1/1 -> Product3/1
  Constant2/1 -> Product1/2
  T/1 -> Product2/4
  Constant5/1 -> Product2/3
  Constant4/1 -> Product2/2

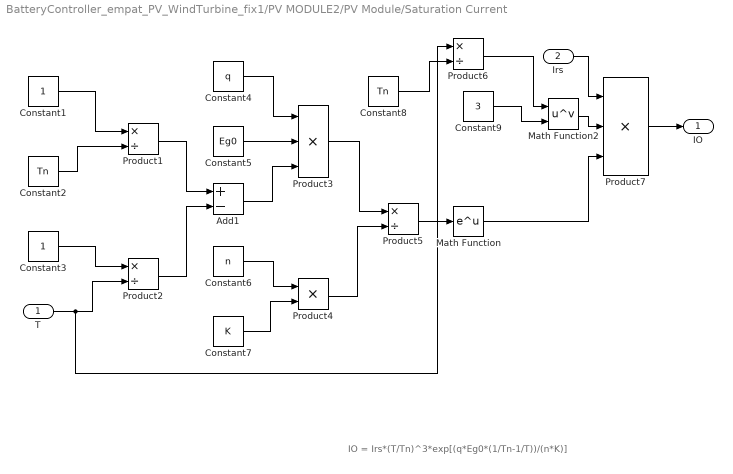
== system BatteryController_empat_PV_WindTurbine_fix1/PV MODULE2/PV Module/Saturation Current ==
  note: IO = Irs*(T/Tn)^3*exp[(q*Eg0*(1/Tn-1/T))/(n*K)]
  T : Inport
  Irs : Inport  Port=2
  Add1 : Sum  Inputs=+-
  Constant1 : Constant
  Constant2 : Constant  Value=Tn
  Constant3 : Constant
  Constant4 : Constant  Value=q
  Constant5 : Constant  Value=Eg0
  Constant6 : Constant  Value=n
  Constant7 : Constant  Value=K
  Constant8 : Constant  Value=Tn
  Constant9 : Constant  Value=3
  Math Function : Math  SaturateOnIntegerOverflow=on
  Math Function2 : Math  Operator=pow  SaturateOnIntegerOverflow=on
  Product{1..2,5..6} (4 alike) : Product  Inputs=*/
  Product3 : Product  Inputs=3
  Product4 : Product
  Product7 : Product  Inputs=3
  IO : Outport
  wires:
  Product7/1 -> IO/1
  Product4/1 -> Product5/2
  Product5/1 -> Math Function/1
  Math Function2/1 -> Product7/2
  Constant2/1 -> Product1/2
  Add1/1 -> Product3/3
  Constant5/1 -> Product3/2
  Constant7/1 -> Product4/2
  Constant4/1 -> Product3/1
  Constant8/1 -> Product6/2
  Product2/1 -> Add1/2
  T/1 -> Product6/1, Product2/2
  Constant1/1 -> Product1/1
  Math Function/1 -> Product7/3
  Product6/1 -> Math Function2/1
  Constant9/1 -> Math Function2/2
  Irs/1 -> Product7/1
  Constant3/1 -> Product2/1
  Product3/1 -> Product5/1
  Constant6/1 -> Product4/1
  Product1/1 -> Add1/1

== system BatteryController_empat_PV_WindTurbine_fix1/PV MODULE2/PV Module/Shunt Current ==
  note: Ish=(V+I*Rs)/Rsh
  V : Inport
  I : Inport  Port=2
  Add1 : Sum
  Constant1 : Constant  Value=Rs
  Constant2 : Constant  Value=Rsh
  Product1 : Product  Inputs=**
  Product2 : Product  Inputs=*/
  Ish : Outport
  wires:
  I/1 -> Product1/1
  Constant1/1 -> Product1/2
  Constant2/1 -> Product2/2
  Add1/1 -> Product2/1
  Product1/1 -> Add1/1
  Product2/1 -> Ish/1
  V/1 -> Add1/2

== system BatteryController_empat_PV_WindTurbine_fix1/PV MODULE3/PV Module/Photo Current ==
  note: Iph=[Isc + {ki*(T-298)}]*G/1000
  T : Inport
  G : Inport  Port=2
  Add1 : Sum  Inputs=+-
  Add2 : Sum  Inputs=+-
  Constant1 : Constant  Value=298
  Constant2 : Constant  Value=ki
  Constant3 : Constant  Value=Isc
  Constant4 : Constant  Value=1000
  Product1 : Product
  Product2 : Product
  Product3 : Product  Inputs=*/
  Iph : Outport
  wires:
  Add2/1 -> Product2/2
  Product3/1 -> Iph/1
  Constant4/1 -> Product3/2
  Constant1/1 -> Add1/2
  Product2/1 -> Product3/1
  G/1 -> Product2/1
  Constant2/1 -> Product1/2
  Product1/1 -> Add2/2
  Add1/1 -> Product1/1
  T/1 -> Add1/1
  Constant3/1 -> Add2/1

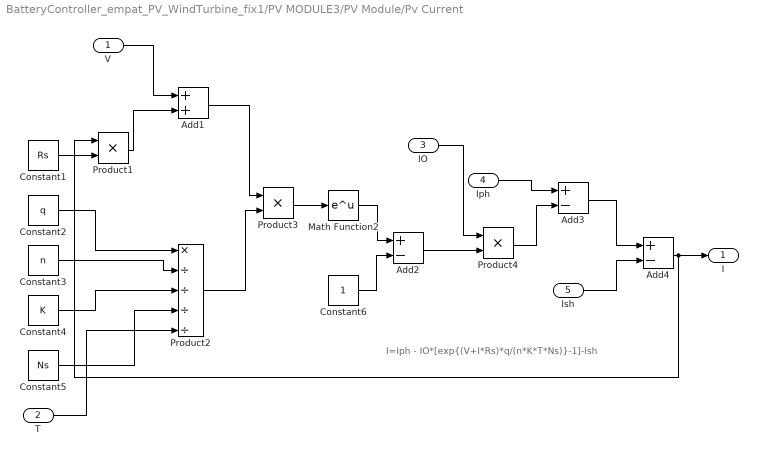
== system BatteryController_empat_PV_WindTurbine_fix1/PV MODULE3/PV Module/Pv Current ==
  note: I=Iph - IO*[exp{(V+I*Rs)*q/(n*K*T*Ns)}-1]-Ish
  V : Inport
  T : Inport  Port=2
  IO : Inport  Port=3
  Iph : Inport  Port=4
  Ish : Inport  Port=5
  Add1 : Sum
  Add2 : Sum  Inputs=+-
  Add3 : Sum  Inputs=+-
  Add4 : Sum  Inputs=+-
  Constant1 : Constant  Value=Rs
  Constant2 : Constant  Value=q
  Constant3 : Constant  Value=n
  Constant4 : Constant  Value=K
  Constant5 : Constant  Value=Ns
  Constant6 : Constant
  Math Function2 : Math  SaturateOnIntegerOverflow=on
  Product1 : Product
  Product2 : Product  Inputs=*////
  Product3 : Product
  Product4 : Product
  I : Outport
  wires:
  Constant3/1 -> Product2/2
  Constant4/1 -> Product2/3
  Add2/1 -> Product4/2
  Add3/1 -> Add4/1
  Constant5/1 -> Product2/4
  Iph/1 -> Add3/1
  Product1/1 -> Add1/2
  Product2/1 -> Product3/2
  T/1 -> Product2/5
  Product3/1 -> Math Function2/1
  Math Function2/1 -> Add2/1
  Add1/1 -> Product3/1
  Constant2/1 -> Product2/1
  V/1 -> Add1/1
  IO/1 -> Product4/1
  Constant6/1 -> Add2/2
  Ish/1 -> Add4/2
  Add4/1 -> I/1, Product1/1
  Product4/1 -> Add3/2
  Constant1/1 -> Product1/2

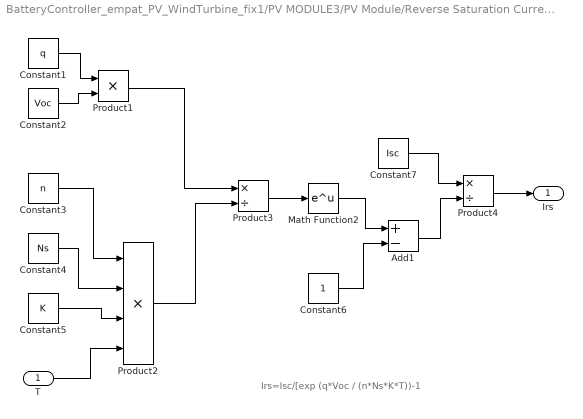
== system BatteryController_empat_PV_WindTurbine_fix1/PV MODULE3/PV Module/Reverse Saturation Current ==
  note: Irs=Isc/[exp (q*Voc / (n*Ns*K*T))-1
  T : Inport
  Add1 : Sum  Inputs=+-
  Constant1 : Constant  Value=q
  Constant2 : Constant  Value=Voc
  Constant3 : Constant  Value=n
  Constant4 : Constant  Value=Ns
  Constant5 : Constant  Value=K
  Constant6 : Constant
  Constant7 : Constant  Value=Isc
  Math Function2 : Math  SaturateOnIntegerOverflow=on
  Product1 : Product
  Product2 : Product  Inputs=4
  Product3 : Product  Inputs=*/
  Product4 : Product  Inputs=*/
  Irs : Outport
  wires:
  Product4/1 -> Irs/1
  Constant1/1 -> Product1/1
  Math Function2/1 -> Add1/1
  Constant6/1 -> Add1/2
  Constant3/1 -> Product2/1
  Add1/1 -> Product4/2
  Product2/1 -> Product3/2
  Constant7/1 -> Product4/1
  Product3/1 -> Math Function2/1
  Product1/1 -> Product3/1
  Constant2/1 -> Product1/2
  T/1 -> Product2/4
  Constant5/1 -> Product2/3
  Constant4/1 -> Product2/2

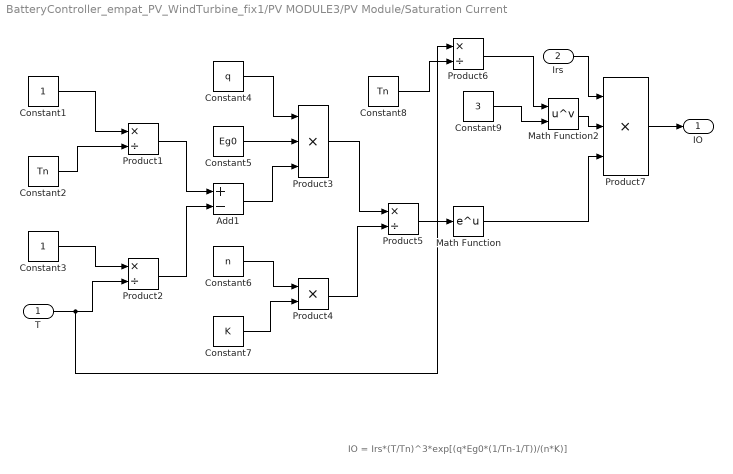
== system BatteryController_empat_PV_WindTurbine_fix1/PV MODULE3/PV Module/Saturation Current ==
  note: IO = Irs*(T/Tn)^3*exp[(q*Eg0*(1/Tn-1/T))/(n*K)]
  T : Inport
  Irs : Inport  Port=2
  Add1 : Sum  Inputs=+-
  Constant1 : Constant
  Constant2 : Constant  Value=Tn
  Constant3 : Constant
  Constant4 : Constant  Value=q
  Constant5 : Constant  Value=Eg0
  Constant6 : Constant  Value=n
  Constant7 : Constant  Value=K
  Constant8 : Constant  Value=Tn
  Constant9 : Constant  Value=3
  Math Function : Math  SaturateOnIntegerOverflow=on
  Math Function2 : Math  Operator=pow  SaturateOnIntegerOverflow=on
  Product{1..2,5..6} (4 alike) : Product  Inputs=*/
  Product3 : Product  Inputs=3
  Product4 : Product
  Product7 : Product  Inputs=3
  IO : Outport
  wires:
  Product7/1 -> IO/1
  Product4/1 -> Product5/2
  Product5/1 -> Math Function/1
  Math Function2/1 -> Product7/2
  Constant2/1 -> Product1/2
  Add1/1 -> Product3/3
  Constant5/1 -> Product3/2
  Constant7/1 -> Product4/2
  Constant4/1 -> Product3/1
  Constant8/1 -> Product6/2
  Product2/1 -> Add1/2
  T/1 -> Product6/1, Product2/2
  Constant1/1 -> Product1/1
  Math Function/1 -> Product7/3
  Product6/1 -> Math Function2/1
  Constant9/1 -> Math Function2/2
  Irs/1 -> Product7/1
  Constant3/1 -> Product2/1
  Product3/1 -> Product5/1
  Constant6/1 -> Product4/1
  Product1/1 -> Add1/1

== system BatteryController_empat_PV_WindTurbine_fix1/PV MODULE3/PV Module/Shunt Current ==
  note: Ish=(V+I*Rs)/Rsh
  V : Inport
  I : Inport  Port=2
  Add1 : Sum
  Constant1 : Constant  Value=Rs
  Constant2 : Constant  Value=Rsh
  Product1 : Product  Inputs=**
  Product2 : Product  Inputs=*/
  Ish : Outport
  wires:
  I/1 -> Product1/1
  Constant1/1 -> Product1/2
  Constant2/1 -> Product2/2
  Add1/1 -> Product2/1
  Product1/1 -> Add1/1
  Product2/1 -> Ish/1
  V/1 -> Add1/2

== system BatteryController_empat_PV_WindTurbine_fix1/PV MODULE4/PV Module/Photo Current ==
  note: Iph=[Isc + {ki*(T-298)}]*G/1000
  T : Inport
  G : Inport  Port=2
  Add1 : Sum  Inputs=+-
  Add2 : Sum  Inputs=+-
  Constant1 : Constant  Value=298
  Constant2 : Constant  Value=ki
  Constant3 : Constant  Value=Isc
  Constant4 : Constant  Value=1000
  Product1 : Product
  Product2 : Product
  Product3 : Product  Inputs=*/
  Iph : Outport
  wires:
  Add2/1 -> Product2/2
  Product3/1 -> Iph/1
  Constant4/1 -> Product3/2
  Constant1/1 -> Add1/2
  Product2/1 -> Product3/1
  G/1 -> Product2/1
  Constant2/1 -> Product1/2
  Product1/1 -> Add2/2
  Add1/1 -> Product1/1
  T/1 -> Add1/1
  Constant3/1 -> Add2/1

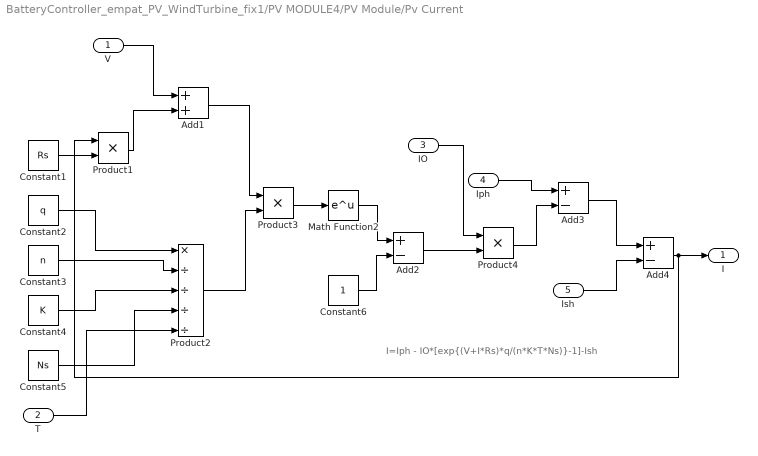
== system BatteryController_empat_PV_WindTurbine_fix1/PV MODULE4/PV Module/Pv Current ==
  note: I=Iph - IO*[exp{(V+I*Rs)*q/(n*K*T*Ns)}-1]-Ish
  V : Inport
  T : Inport  Port=2
  IO : Inport  Port=3
  Iph : Inport  Port=4
  Ish : Inport  Port=5
  Add1 : Sum
  Add2 : Sum  Inputs=+-
  Add3 : Sum  Inputs=+-
  Add4 : Sum  Inputs=+-
  Constant1 : Constant  Value=Rs
  Constant2 : Constant  Value=q
  Constant3 : Constant  Value=n
  Constant4 : Constant  Value=K
  Constant5 : Constant  Value=Ns
  Constant6 : Constant
  Math Function2 : Math  SaturateOnIntegerOverflow=on
  Product1 : Product
  Product2 : Product  Inputs=*////
  Product3 : Product
  Product4 : Product
  I : Outport
  wires:
  Constant3/1 -> Product2/2
  Constant4/1 -> Product2/3
  Add2/1 -> Product4/2
  Add3/1 -> Add4/1
  Constant5/1 -> Product2/4
  Iph/1 -> Add3/1
  Product1/1 -> Add1/2
  Product2/1 -> Product3/2
  T/1 -> Product2/5
  Product3/1 -> Math Function2/1
  Math Function2/1 -> Add2/1
  Add1/1 -> Product3/1
  Constant2/1 -> Product2/1
  V/1 -> Add1/1
  IO/1 -> Product4/1
  Constant6/1 -> Add2/2
  Ish/1 -> Add4/2
  Add4/1 -> I/1, Product1/1
  Product4/1 -> Add3/2
  Constant1/1 -> Product1/2

== system BatteryController_empat_PV_WindTurbine_fix1/PV MODULE4/PV Module/Reverse Saturation Current ==
  note: Irs=Isc/[exp (q*Voc / (n*Ns*K*T))-1
  T : Inport
  Add1 : Sum  Inputs=+-
  Constant1 : Constant  Value=q
  Constant2 : Constant  Value=Voc
  Constant3 : Constant  Value=n
  Constant4 : Constant  Value=Ns
  Constant5 : Constant  Value=K
  Constant6 : Constant
  Constant7 : Constant  Value=Isc
  Math Function2 : Math  SaturateOnIntegerOverflow=on
  Product1 : Product
  Product2 : Product  Inputs=4
  Product3 : Product  Inputs=*/
  Product4 : Product  Inputs=*/
  Irs : Outport
  wires:
  Product4/1 -> Irs/1
  Constant1/1 -> Product1/1
  Math Function2/1 -> Add1/1
  Constant6/1 -> Add1/2
  Constant3/1 -> Product2/1
  Add1/1 -> Product4/2
  Product2/1 -> Product3/2
  Constant7/1 -> Product4/1
  Product3/1 -> Math Function2/1
  Product1/1 -> Product3/1
  Constant2/1 -> Product1/2
  T/1 -> Product2/4
  Constant5/1 -> Product2/3
  Constant4/1 -> Product2/2

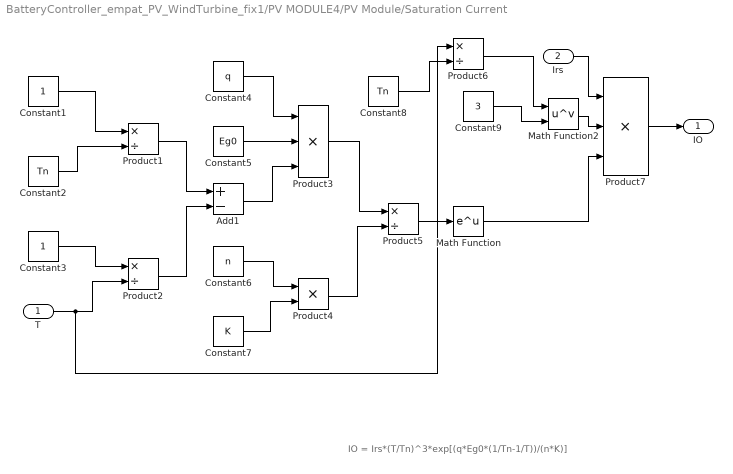
== system BatteryController_empat_PV_WindTurbine_fix1/PV MODULE4/PV Module/Saturation Current ==
  note: IO = Irs*(T/Tn)^3*exp[(q*Eg0*(1/Tn-1/T))/(n*K)]
  T : Inport
  Irs : Inport  Port=2
  Add1 : Sum  Inputs=+-
  Constant1 : Constant
  Constant2 : Constant  Value=Tn
  Constant3 : Constant
  Constant4 : Constant  Value=q
  Constant5 : Constant  Value=Eg0
  Constant6 : Constant  Value=n
  Constant7 : Constant  Value=K
  Constant8 : Constant  Value=Tn
  Constant9 : Constant  Value=3
  Math Function : Math  SaturateOnIntegerOverflow=on
  Math Function2 : Math  Operator=pow  SaturateOnIntegerOverflow=on
  Product{1..2,5..6} (4 alike) : Product  Inputs=*/
  Product3 : Product  Inputs=3
  Product4 : Product
  Product7 : Product  Inputs=3
  IO : Outport
  wires:
  Product7/1 -> IO/1
  Product4/1 -> Product5/2
  Product5/1 -> Math Function/1
  Math Function2/1 -> Product7/2
  Constant2/1 -> Product1/2
  Add1/1 -> Product3/3
  Constant5/1 -> Product3/2
  Constant7/1 -> Product4/2
  Constant4/1 -> Product3/1
  Constant8/1 -> Product6/2
  Product2/1 -> Add1/2
  T/1 -> Product6/1, Product2/2
  Constant1/1 -> Product1/1
  Math Function/1 -> Product7/3
  Product6/1 -> Math Function2/1
  Constant9/1 -> Math Function2/2
  Irs/1 -> Product7/1
  Constant3/1 -> Product2/1
  Product3/1 -> Product5/1
  Constant6/1 -> Product4/1
  Product1/1 -> Add1/1

== system BatteryController_empat_PV_WindTurbine_fix1/PV MODULE4/PV Module/Shunt Current ==
  note: Ish=(V+I*Rs)/Rsh
  V : Inport
  I : Inport  Port=2
  Add1 : Sum
  Constant1 : Constant  Value=Rs
  Constant2 : Constant  Value=Rsh
  Product1 : Product  Inputs=**
  Product2 : Product  Inputs=*/
  Ish : Outport
  wires:
  I/1 -> Product1/1
  Constant1/1 -> Product1/2
  Constant2/1 -> Product2/2
  Add1/1 -> Product2/1
  Product1/1 -> Add1/1
  Product2/1 -> Ish/1
  V/1 -> Add1/2
